simulink model "ekf"  (R2018b)
settings: Solver=ode5  StartTime=0.0  StopTime=15  FixedStep=0.1  MaxStep=0.1  RelTol=1e-3  AbsTol=1e-6
StartFcn:
  | clear radarLogsOut
StopFcn:
  | aero_radplot;
model workspace (MATLAB code in the model file):
  | g = 32.2;    % Acceleration due to gravity (ft/sec^2)
  | tauc = 5;    % Correlation time of aircraft cross axis acceleration
  | tauT = 4;    % Correlation time of aircraft thrust axis acceleration
  | Speed = 400; % Initial speed of aircraft in y direction feet/sec
  | deltat = 1;  % Radar update rate (also hard-coded in extkalman.m)
libraries: simulink x3
CloseFcn:
  | h=findobj('type','figure');if ~isempty(h);close(h);end
  | clear radarLogsOut
  | clear h;
Description:
  | Radar Tracking Using MATLAB Function Block
  | 
  | This example shows how to use an extended Kalman filter with the
  | MATLAB(R) Function block in Simulink(R) to estimate an aircraft's
  | position from radar measurements. The filter implementation is found in the
  | MATLAB Function block, the contents of which are stored in the
  | Simulink model itself.
  | 
  | At the end of the simulation, three figures display the following information: the
  | actual trajectory compared to the estimated trajectory; the estimation residual
  | for range; and the actual, measured, and estimated positions.
settings Model: ExtModeTrigMode=oneshot  ExtModeArmWhenConnect=off  ExtModeAutoUpdateStatusClock=off  Creator=The MathWorks, Inc.  LastModifiedBy=1star
settings SolverCC: AutoScaleAbsTol=off
settings DataIOCC: SaveFormat=Array  SaveOutput=off  SaveTime=off  TimeSaveName=t_sim  SignalLoggingName=radarLogsOut
settings OptimizationCC: DefaultParameterBehavior=Inlined  InlineInvariantSignals=on  ExpressionDepthLimit=2147483647  StateBitsets=on  DataBitsets=on  ZeroExternalMemoryAtStartup=off  ZeroInternalMemoryAtStartup=off  NoFixptDivByZeroProtection=on  LifeSpan=1  BufferReusableBoundary=off
settings DebuggingCC: SaveWithParameterizedLinksMsg=none  CheckExecutionContextPreStartOutputMsg=on  CheckExecutionContextRuntimeOutputMsg=on  SignalResolutionControl=TryResolveAllWithWarning  MultiTaskDSMMsg=warning  MultiTaskCondExecSysMsg=none  FcnCallInpInsideContextMsg=warning  StateNameClashWarn=warning  SFUnexpectedBacktrackingDiag=warning  SFNoUnconditionalDefaultTransitionDiag=warning  SFExecutionAtInitializationDiag=none
settings HardwareCC: ProdBitPerPointer=32  ProdBitPerSizeT=32  ProdBitPerPtrDiffT=32  ProdLargestAtomicFloat=None  ProdIntDivRoundTo=Undefined  ProdEndianess=Unspecified  ProdWordSize=32  ProdHWDeviceType=32-bit Generic
settings ModelReferenceCC: PropagateSignalLabelsOutOfModel=off
settings SFSimCC: SimUseLocalCustomCode=off  SimParseCustomCode=off  MATLABDynamicMemAlloc=off
settings RTWCC: SystemTargetFile=ert.tlc  TLCOptions=-p0 -aWarnNonSaturatedBlocks=0  TemplateMakefile=ert_default_tmf  Description=RTW Embedded Coder (no auto configuration)  GenerateReport=on  RTWVerbose=off  RTWUseLocalCustomCode=off  IncludeHyperlinkInReport=on  LaunchReport=on
settings CodeAppCC: ForceParamTrailComments=on  IgnoreCustomStorageClasses=off  SimulinkDataObjDesc=on  CustomSymbolStrType=$N$R$M  CustomSymbolStrFcn=$F$N$M  CustomSymbolStrMacro=$N$M  InsertBlockDesc=on  StateflowObjectComments=on  InternalIdentifier=Classic
settings ERTTargetCC: TargetFcnLib=ansi_tfl_tmw.mat  MultiwordLength=2048  GenerateSampleERTMain=on  IncludeMdlTerminateFcn=off  SupportComplex=off  SupportContinuousTime=on  SupportNonInlinedSFcns=on  InlinedParameterPlacement=NonHierarchical  ERTCustomFileTemplate=example_file_process.tlc  ConvertIfToSwitch=off  SuppressUnreachableDefaultCases=off
settings ConfigComp: CovMetricSettings=d  CovHtmlReporting=on  CovSaveCumulativeToWorkspaceVar=on  CovSaveSingleToWorkspaceVar=on  CovExternalEMLEnable=off

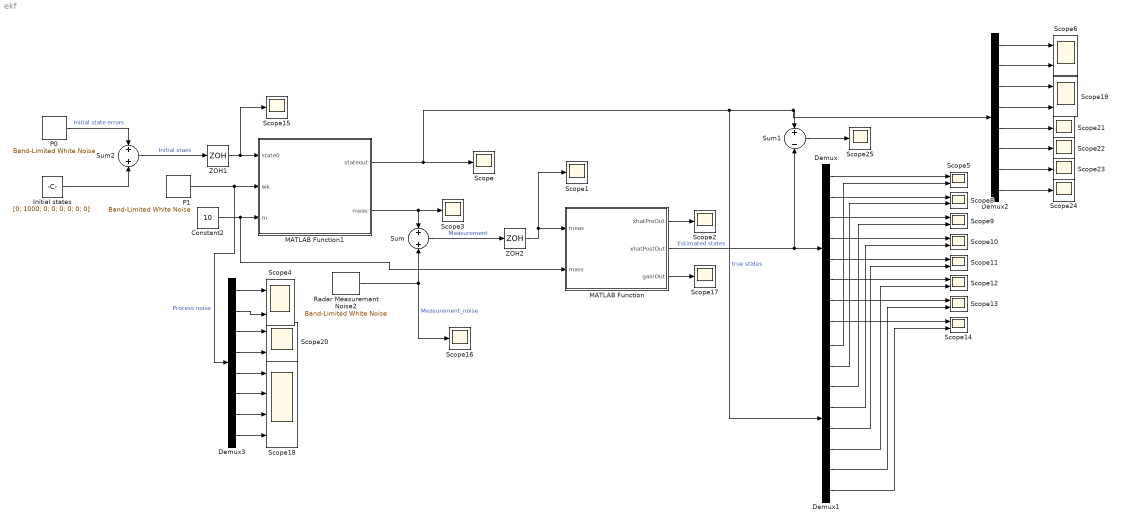
== system ekf ==
  Constant2 : Constant  Value=10  SampleTime=0.1
  Demux{,1..3} (4 alike) : Demux  Outputs=8
  Initial states : Constant  Value=[0; 1000; 0; 0; 0; 0; 0; 0]  SampleTime=deltat
  MATLAB Function : MATLAB Function  TreatAsAtomicUnit=on
  MATLAB Function1 : MATLAB Function  TreatAsAtomicUnit=on
  P0 : simulink/Sources/Band-Limited White Noise  Cov=[100 1000 0.1 10 0.2 15 0.1 900]  Ts=0.1  seed=[52345; 62341; 72341; 82341; 92341; 10341; 11341; 12341]
  P1 : simulink/Sources/Band-Limited White Noise  Cov=[0 0 0 0.2 0 0 0 0]  Ts=0.1  seed=[52345; 62341; 72341; 82341; 92341; 10341; 11341; 12341]
  Radar Measurement Noise2 : simulink/Sources/Band-Limited White Noise  Cov=4  Ts=0.1  seed=[52342]
  Scope{,1..3,15..17,21..25} (12 alike) : Scope
  Scope{4..6,8..14,19..20} (12 alike) : Scope  NumInputPorts=2
  Scope18 : Scope  NumInputPorts=4
  Sum : Sum  Inputs=2  SaturateOnIntegerOverflow=on  InputSameDT=on  OutDataTypeStr=Inherit: Same as first input
  Sum1 : Sum  Inputs=+-  SaturateOnIntegerOverflow=on  InputSameDT=on  OutDataTypeStr=Inherit: Same as first input
  Sum2 : Sum  SaturateOnIntegerOverflow=on  InputSameDT=on  OutDataTypeStr=Inherit: Same as first input
  ZOH1 : ZeroOrderHold  SampleTime=0.1
  ZOH2 : ZeroOrderHold  SampleTime=0.5
  wires:
  MATLAB Function/2(xhatPostOut) -> Sum1/2, Demux/1  "Estimated states"
  MATLAB Function1/2(meas) -> Sum/1, Scope3/1
  Radar Measurement Noise2/1 -> Scope16/1, Sum/2  "Measurement_noise"
  Sum/1 -> ZOH2/1  "Measurement"
  ZOH1/1 -> Scope15/1, MATLAB Function1/1(state0)
  P1/1 -> MATLAB Function1/2(wk), Demux3/1  "Process noise"
  Constant2/1 -> MATLAB Function/2(mass), MATLAB Function1/3(m)
  ZOH2/1 -> MATLAB Function/1(meas), Scope1/1
  Initial states/1 -> Sum2/2
  P0/1 -> Sum2/1  "Initial state errors"
  Sum2/1 -> ZOH1/1  "Initial staes"
  Demux/1 -> Scope5/1
  Demux/2 -> Scope8/1
  Demux/3 -> Scope9/1
  Demux/4 -> Scope10/1
  Demux/5 -> Scope11/1
  Demux/6 -> Scope12/1
  Demux/7 -> Scope13/1
  Demux/8 -> Scope14/1
  Demux1/7 -> Scope13/2
  Demux1/3 -> Scope9/2
  Demux1/6 -> Scope12/2
  Demux1/8 -> Scope14/2
  MATLAB Function1/1(stateout) -> Scope/1, Demux2/1, Sum1/1, Demux1/1  "true states"
  Demux1/2 -> Scope8/2
  Demux1/5 -> Scope11/2
  Demux1/4 -> Scope10/2
  Demux1/1 -> Scope5/2
  MATLAB Function/3(gainOut) -> Scope17/1
  Demux2/1 -> Scope6/1
  Demux2/3 -> Scope19/1
  Demux2/4 -> Scope19/2
  Demux2/5 -> Scope21/1
  Demux2/6 -> Scope22/1
  Demux2/8 -> Scope24/1
  Demux2/7 -> Scope23/1
  Sum1/1 -> Scope25/1
  Demux2/2 -> Scope6/2
  Demux3/1 -> Scope4/1
  Demux3/2 -> Scope4/2
  Demux3/3 -> Scope20/1
  Demux3/4 -> Scope20/2
  Demux3/5 -> Scope18/1
  Demux3/6 -> Scope18/2
  Demux3/7 -> Scope18/3
  Demux3/8 -> Scope18/4
  MATLAB Function/1(xhatPreOut) -> Scope2/1

== matlab function ekf/MATLAB Function1 ==
  data: state0 input double; wk input; m input; stateout output double; meas output
function [stateout, meas]  = Envrionment(state0, wk, m)

% Initialization
deltat = 0.1;
g=9.836;
persistent state;

if isempty(state)
    state = state0;
end
 
h_ = 2;
bet_ = 150;
rho0_ = 1.225;
kp_ = 9200;
% 

ry = state(2);
vy = state(4);

deltabet = state(6);
deltarho = state(7);
deltakp = state(8);
% 
bet=bet_+deltabet;
rho0=rho0_+deltarho;
kp=kp_+deltakp;
% 
alpha = rho0*exp(-ry/kp)*vy*vy/(2*m*bet);
% 
phi = [1 0 deltat 0 0 0 0 0; 0 1 0 deltat 0 0 0 0; 0 0 1 0 0 0 0 0; 0 -alpha*deltat/kp 0 1+rho0*exp(-ry/kp)*vy/(m*bet)*deltat 0 -alpha/bet*deltat alpha/rho0*deltat ry*alpha*deltat/(kp*kp);
    0 0 0 0 1 0 0 0; 0 0 0 0 0 1 0 0; 0 0 0 0 0 0 1 0; 0 0 0 0 0 0 0 1];
u = [0; -g*deltat*deltat/2; 0; -g*deltat*(1+rho0*exp(-ry/kp)*vy/(2*m*bet)); 0; 0; 0; 0];

state = phi*state + u + wk;
rx=state(1);
ry=state(2);
deltah=state(5);
y=sqrt(rx^2+(ry-h_-deltah)^2);
% y=ry;

meas = y;

stateout = state;

== matlab function ekf/MATLAB Function ==
  data: meas input double; xhatPreOut output; xhatPostOut output double; gainOut output; mass input
function [xhatPreOut, xhatPostOut,gainOut] = EXTKALMAN(meas,mass)

%input param
    %meas: measurement from radar.ie.the distance from radar to falling body
    %mass: mass of falling body
persistent P_post;
persistent xhat_post

%Initialize simulation parameters.
delta_t=0.5;         %Updating time of EKF.
g=9.836;             %gravity acceleration   
m = mass;            %mass of falling body  
h_ = 2;              %init value of height of radar
bet_ = 150;          %init value of ballistic coefficient of the falling body
rho0_ = 1.225;       %init value of the atmospheric density at sea level
kp_ = 9200;

%step1. Initialize the state

if isempty(P_post)      %if simulation is started initialize the covairance matrix of estimates
    xhat_post = [0; 1000; 0; 0; 0; 0; 0; 0];
    P_post = zeros(8);
    P_post(1)=100;
    P_post(2)=1000;    
end

%  Compute Phi, Q, and R 

%get params for computaion of Phi from the previous post estimates.
ry = xhat_post(2);
vy = xhat_post(4);
deltabet = xhat_post(6);
bet=bet_+deltabet;
deltarho = xhat_post(7);
rho0=rho0_+deltarho;
deltakp = xhat_post(8);
kp=kp_+deltakp;

alpha = rho0*exp(-ry/kp)*vy*vy/(2*m*bet);   %params to calculate Phi

Phi = [1 0 delta_t 0 0 0 0 0; 0 1 0 delta_t 0 0 0 0; 0 0 1 0 0 0 0 0; 0 -alpha*delta_t/kp 0 1+rho0*exp(-ry/kp)*vy/(m*bet)*delta_t 0 -alpha/bet*delta_t alpha/rho0*delta_t ry*alpha*delta_t/(kp*kp);
    0 0 0 0 1 0 0 0; 0 0 0 0 0 1 0 0; 0 0 0 0 0 0 1 0; 0 0 0 0 0 0 0 1];
Q =  diag([0 0 0 10 0 0 0 0 ]);
R =  diag(4);

%Step 2. Propagate the estimate:

u = [0; -g*delta_t*delta_t/2; 0; -g*delta_t*(1+rho0*exp(-ry/kp)*vy/(2*m*bet)); 0; 0; 0; 0];
xhat_pre = Phi*xhat_post+u;                 %propagate estimate from previous post estimates to current pre estimates.
P_pre = Phi*P_post*Phi' + Q;                %calculate the covariance matrix for current pre estimates

%Step 3: Update the states

rx_pre=xhat_pre(1);            
ry_pre=xhat_pre(2);
h_pre=h_+xhat_pre(5);
rm=sqrt(rx_pre^2+(ry_pre-h_pre)^2);         %get the length from radar to object

yhat_pre=rm;                                %get the measures

H1=rx_pre/rm;
H2=(ry_pre-h_pre)/rm;
H5=-H2;
H = [H1 H2 0 0 H5 0 0 0];   

Kk = P_pre*H'/(H*P_pre*H'+ R);              %Compute Kalman Gain:
xhat_post = xhat_pre + Kk*(meas - yhat_pre);    %pdate estimate
P_post = (eye(8)-Kk*H)*P_pre;               %Update Covariance Matrix

%output the pre estimates,post estimates and kalman gain
xhatPreOut = xhat_pre;                      %Output the pre estimates.
xhatPostOut = xhat_post;                    %output post estimates.
gainOut = Kk;
